simulink model "vie"  (Simulink 7.9)
settings: Solver=ode45  StartTime=0.0  StopTime=10.0  RelTol=1e-3
values from neighbouring files (symbols this model uses):
  Ta = 0.38    [parameters.m]
settings Model: Creator=dede  LastModifiedBy=dede

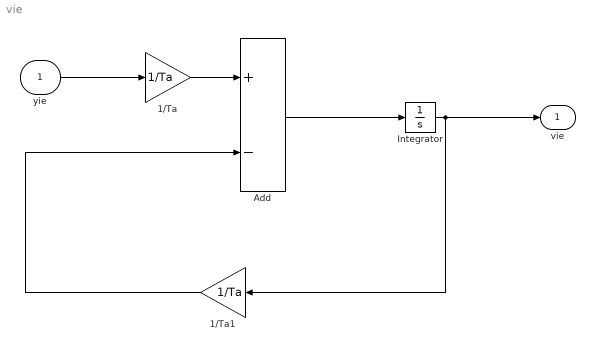
== system vie ==
  yie : Inport
  1/Ta : Gain  Gain=1/Ta
  1/Ta1 : Gain  Gain=1/Ta
  Add : Sum  Inputs=+-
  Integrator : Integrator
  vie : Outport
  wires:
  yie/1 -> 1/Ta/1
  1/Ta/1 -> Add/1
  Add/1 -> Integrator/1
  Integrator/1 -> 1/Ta1/1, vie/1
  1/Ta1/1 -> Add/2
